simulink model "B2_IEEE_13_bus"  (R2022b)
settings: Solver=ode4  StartTime=0.0  StopTime=tend  FixedStep=ts  MaxStep=0.04  RelTol=1e-3
undefined symbols (not defined in the file): C, C_601, C_602, C_603, C_604, C_605, C_606, C_607, C_bc_ESS, C_bc_PV, C_bc_SC, C_SC_set, Cf, f0, fc, fc1, ft2km, fv, Gf, Idcbase, Ilim, J, Ki_c1, Ki_v, Kp_c1, Kp_v, L_601, L_602, L_603, L_604, L_605, L_606, L_607, L_bc_ESS, L_bc_PV, L_bc_SC, L_line_ESS, L_line_PV, Lf, Pnom, Pset_ESS, Pset_inv, Pset_load, Pset_PV, Pset_SC, Qset_inv, R_601, R_602, R_603, R_604, R_605, R_606, R_607, R_bc_ESS, R_bc_PV, R_bc_SC, R_line_ESS, R_line_PV, R_line_SC, Rf ... (+23)
libraries: spsSeriesRLCBranchLib x12, spsLoadFlowBusLib x12, spsPiSectionLineLib x9, spsThreePhaseVIMeasurementLib x8, spsVoltageMeasurementLib x8, cstblocks x8, spsThreePhaseSeriesRLCLoadLib x7, spsCurrentMeasurementLib x6, simulink_extras x6, spsGroundLib x6, spsMultimeterLib x6, spsPowerLib x6
(part 2 of 2)

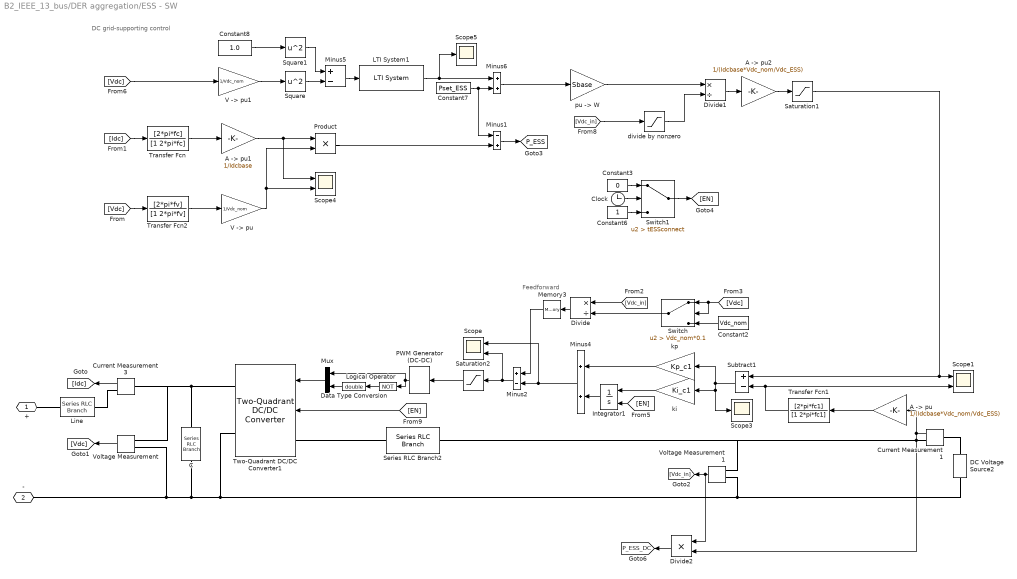
== system B2_IEEE_13_bus/DER aggregation/ESS - SW ==
  note: Feedforward
  note: DC grid-supporting control
  "A -> pu" : Gain  Gain=1/(Idcbase*Vdc_nom/Vdc_ESS)
  "A -> pu1" : Gain  Gain=1/Idcbase
  "A -> pu2" : Gain  Gain=1/(Idcbase*Vdc_nom/Vdc_ESS)
  C : spsSeriesRLCBranchLib/Series RLC Branch  LConnTagsString=__new0  RConnTagsString=__new0  BranchType=C  Resistance=0.001  Inductance=L_line_PV  SetiL0=off  InitialCurrent=0  Capacitance=C_bc_ESS  Setx0=on  InitialVoltage=Vdc_nom  Measurements=None
  Clock : Clock
  Constant2 : Constant  Value=Vdc_nom
  Constant3 : Constant  Value=0
  Constant6 : Constant
  Constant7 : Constant  Value=Pset_ESS
  Constant8 : Constant  Value=1.0
  Current Measurement1 : spsCurrentMeasurementLib/Current Measurement  PhasorSimulation=off  OutputType=Complex  PSBequivalent=0
  Current Measurement3 : spsCurrentMeasurementLib/Current Measurement  PhasorSimulation=off  OutputType=Complex  PSBequivalent=0
  DC Voltage Source2 : spsDCVoltageSourceLib/DC Voltage Source  Amplitude=Vdc_ESS  Measurements=None
  Data Type Conversion : DataTypeConversion  OutDataTypeStr=double  SaturateOnIntegerOverflow=off  RndMeth=Floor
  Divide : Product  Inputs=*/
  Divide1 : Product  Inputs=*/
  Divide2 : Product  Inputs=**
  Integrator1 : Integrator  ExternalReset=level hold  LimitOutput=on  UpperSaturationLimit=1  LowerSaturationLimit=-1
  LTI System1 : cstblocks/LTI System  sys=T_ESS1  IC=[]
  Line : spsSeriesRLCBranchLib/Series RLC Branch  LConnTagsString=__new0  RConnTagsString=__new0  BranchType=R  Resistance=R_line_ESS  Inductance=L_line_ESS  SetiL0=off  InitialCurrent=0  Capacitance=1e-6  Setx0=off  InitialVoltage=0  Measurements=None
  Logical Operator : Logic  Operator=NOT  AllPortsSameDT=off  OutDataTypeStr=boolean
  Memory3 : Memory
  Minus1 : Sum  Inputs=-+
  Minus2 : Sum  Inputs=+-
  Minus4 : Sum
  Minus5 : Sum  Inputs=+-
  Minus6 : Sum
  Mux : Mux  Inputs=2
  PWM Generator (DC-DC) : spsPWMGeneratorDCDCLib/PWM Generator (DC-DC)  Fsw=fw  Ts=0
  Product : Product
  Saturation1 : Saturate  UpperLimit=1.0  LowerLimit=-1.0
  Saturation2 : Saturate  UpperLimit=1  LowerLimit=0
  Scope : Scope  NumInputPorts=2
  Scope1 : Scope  NumInputPorts=2
  Scope3 : Scope
  Scope4 : Scope  NumInputPorts=2
  Scope5 : Scope
  Series RLC Branch2 : spsSeriesRLCBranchLib/Series RLC Branch  LConnTagsString=__new0  RConnTagsString=__new0  BranchType=RL  Resistance=R_bc_ESS  Inductance=L_bc_ESS  SetiL0=off  InitialCurrent=Pset_ESS*Idcbase*Vdc_nom/Vdc_PV  Capacitance=1e-6  Setx0=off  InitialVoltage=0  Measurements=None
  Square : Math  Operator=square
  Square1 : Math  Operator=square
  Subtract1 : Sum  Inputs=+-
  Switch : Switch  Criteria=u2 > Threshold  Threshold=Vdc_nom*0.1  SaturateOnIntegerOverflow=off  InputSameDT=off
  Switch1 : Switch  Criteria=u2 > Threshold  Threshold=tESSconnect  SaturateOnIntegerOverflow=off  InputSameDT=off
  Transfer Fcn : TransferFcn  Numerator=[2*pi*fc]  Denominator=[1 2*pi*fc]
  Transfer Fcn1 : TransferFcn  Numerator=[2*pi*fc1]  Denominator=[1 2*pi*fc1]
  Transfer Fcn2 : TransferFcn  Numerator=[2*pi*fv]  Denominator=[1 2*pi*fv]
  Two-Quadrant DC/DC Converter1 : spsTwoQuadrantDCDCConverterLib/Two-Quadrant DC//DC Converter  ModelType=Switching devices  Ron=1e-4  Rs=1e6  Cs=inf  Vforward=[0,0]  Ron_Diode=1e-3  Rs_Diode=1e6  Cs_Diode=inf  Vf_Diode=1e-3  Rs_CurrentSource=inf  Ron_ACsource=1e-3
      settings: LibrarySourceBlock=|
      | sps_lib/Power Electronics/Two-Quadrant
      | DC//DC Converter
  "V -> pu" : Gain  Gain=1/Vdc_nom
  "V -> pu1" : Gain  Gain=1/Vdc_nom
  Voltage Measurement : spsVoltageMeasurementLib/Voltage Measurement  PhasorSimulation=off  OutputType=Complex  PSBequivalent=0
  Voltage Measurement1 : spsVoltageMeasurementLib/Voltage Measurement  PhasorSimulation=off  OutputType=Complex  PSBequivalent=0
  divide by nonzero : Saturate  UpperLimit=1e6  LowerLimit=1e-6
  ki : Gain  Gain=Ki_c1
  kp : Gain  Gain=Kp_c1
  "pu -> W" : Gain  Gain=Sbase
  + : PMIOPort  Side=Left
  - : PMIOPort  Port=2  Side=Right
  tag scope: P_ESS=global, P_ESS_DC=global
  wires:
  Constant6/1 -> Switch1/3
  Switch1/1 -> [EN]
  Clock/1 -> Switch1/2
  Constant3/1 -> Switch1/1
  Minus6/1 -> "pu -> W"/1
  Saturation1/1 -> Scope1/1, Subtract1/1
  Divide1/1 -> "A -> pu2"/1
  "pu -> W"/1 -> Divide1/1
  divide by nonzero/1 -> Divide1/2
  Subtract1/1 -> Scope3/1, ki/1, kp/1
  Memory3/1 -> Minus2/1
  Transfer Fcn2/1 -> "V -> pu"/1
  Transfer Fcn/1 -> "A -> pu1"/1
  Minus2/1 -> Scope/2, Saturation2/1
  Minus4/1 -> Minus2/2, Scope/1
  [Vdc] -> Transfer Fcn2/1
  "A -> pu1"/1 -> Product/1, Scope4/1
  "V -> pu"/1 -> Scope4/2, Product/2
  "V -> pu1"/1 -> Square/1
  [Vdc] -> "V -> pu1"/1
  LTI System1/1 -> Scope5/1, Minus6/1
  Constant7/1 -> Minus6/2, Minus1/1
  Minus5/1 -> LTI System1/1
  Square1/1 -> Minus5/1
  Square/1 -> Minus5/2
  Constant8/1 -> Square1/1
  [EN] -> Integrator1/2
  ki/1 -> Integrator1/1
  Integrator1/1 -> Minus4/2
  kp/1 -> Minus4/1
  "A -> pu2"/1 -> Saturation1/1
  [Vdc] -> Switch/1, Switch/2
  Divide/1 -> Memory3/1
  [Vdc_in] -> Divide/1
  Constant2/1 -> Switch/3
  Switch/1 -> Divide/2
  Product/1 -> Minus1/2
  Transfer Fcn1/1 -> Subtract1/2, Scope1/2
  [EN] -> Two-Quadrant DC/DC Converter1/2
  Current Measurement3/1 -> [Idc]
  Voltage Measurement/1 -> [Vdc]
  [Idc] -> Transfer Fcn/1
  "A -> pu"/1 -> Transfer Fcn1/1
  Minus1/1 -> [P_ESS]
  Saturation2/1 -> PWM Generator (DC-DC)/1
  PWM Generator (DC-DC)/1 -> Mux/1, Logical Operator/1
  Logical Operator/1 -> Data Type Conversion/1
  Data Type Conversion/1 -> Mux/2
  Mux/1 -> Two-Quadrant DC/DC Converter1/1
  [Vdc_in] -> divide by nonzero/1
  Voltage Measurement1/1 -> Divide2/1, [Vdc_in]
  Current Measurement1/1 -> "A -> pu"/1, Divide2/2
  Divide2/1 -> [P_ESS_DC]
  connections:
  Line/LConn1 -- +/RConn1
  C/LConn1 -- Two-Quadrant DC/DC Converter1/RConn1 -- Voltage Measurement/LConn1 -- Current Measurement3/LConn1
  Current Measurement3/RConn1 -- Line/RConn1
  Current Measurement1/RConn1 -- Voltage Measurement1/LConn1 -- Series RLC Branch2/RConn1
  DC Voltage Source2/RConn1 -- Current Measurement1/LConn1
  Two-Quadrant DC/DC Converter1/LConn1 -- Series RLC Branch2/LConn1
  Voltage Measurement/LConn2 -- -/RConn1 -- C/RConn1 -- Two-Quadrant DC/DC Converter1/RConn2 -- DC Voltage Source2/LConn1 -- Voltage Measurement1/LConn2

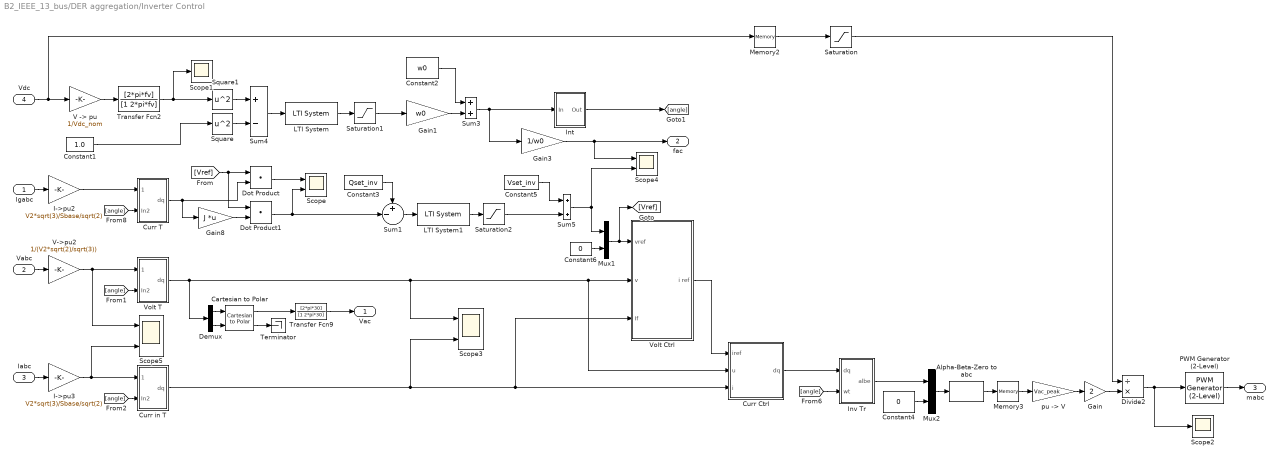
== system B2_IEEE_13_bus/DER aggregation/Inverter Control ==
  Igabc : Inport
  Vabc : Inport  Port=2
  Iabc : Inport  Port=3
  Vdc : Inport  Port=4
  Alpha-Beta-Zero to abc : spsAlphaBetaZerotoabcLib/Alpha-Beta-Zero to abc
  Cartesian to Polar : simulink_extras/Transformations/Cartesian to Polar
  Constant1 : Constant  Value=1.0
  Constant2 : Constant  Value=w0
  Constant3 : Constant  Value=Qset_inv
  Constant4 : Constant  Value=0
  Constant5 : Constant  Value=Vset_inv
  Constant6 : Constant  Value=0
  Curr Ctrl : Subsystem
  Curr T : Subsystem
  Curr in T : Subsystem
  Demux : Demux  Outputs=2
  Divide2 : Product  Inputs=/*
  Dot Product : DotProduct  OutDataTypeStr=Inherit: Inherit via internal rule
  Dot Product1 : DotProduct  OutDataTypeStr=Inherit: Inherit via internal rule
  Gain : Gain  Gain=2
  Gain1 : Gain  Gain=w0
  Gain3 : Gain  Gain=1/w0
  Gain8 : Gain  Gain=J  Multiplication=Matrix(K*u)
  I->pu2 : Gain  Gain=V2*sqrt(3)/Sbase/sqrt(2)  SaturateOnIntegerOverflow=on  OutDataTypeStr=Inherit: Same as input  ParamDataTypeStr=Inherit: Same as input
  I->pu3 : Gain  Gain=V2*sqrt(3)/Sbase/sqrt(2)  SaturateOnIntegerOverflow=on  OutDataTypeStr=Inherit: Same as input  ParamDataTypeStr=Inherit: Same as input
  Int : Subsystem
  Inv Tr : Subsystem
  LTI System : cstblocks/LTI System  sys=T_des_fvdc  IC=[]
  LTI System1 : cstblocks/LTI System  sys=T_des_vq  IC=[]
  Memory2 : Memory
  Memory3 : Memory
  Mux1 : Mux  Inputs=2
  Mux2 : Mux  Inputs=2
  PWM Generator (2-Level) : spsPWMGenerator2LevelLib/PWM Generator (2-Level)  ModulatorType=Three-phase bridge (6 pulses)  ModulatorMode=Unsynchronized  Fc=fw  Pc=90  nF=27  MinMax="[ -1  1 ]"  SamplingTechnique=Natural  ModulatingSignals=off  m=0.8  Freq=60  Phase=0  Ts=0  ShowCarrierOutport=off
  Saturation : Saturate  UpperLimit=Vdc_nom*1.1  LowerLimit=Vdc_nom*0.9
  Saturation1 : Saturate  UpperLimit=0.1  LowerLimit=-0.1
  Saturation2 : Saturate
  Scope{,3..5} (4 alike) : Scope  NumInputPorts=2
  Scope1 : Scope
  Scope2 : Scope
  Square : Math  Operator=square
  Square1 : Math  Operator=square
  Sum1 : Sum  Inputs=+-|
  Sum3 : Sum
  Sum4 : Sum  Inputs=+-
  Sum5 : Sum
  Terminator : Terminator
  Transfer Fcn2 : TransferFcn  Numerator=[2*pi*fv]  Denominator=[1 2*pi*fv]
  Transfer Fcn9 : TransferFcn  Numerator=[2*pi*30]  Denominator=[1 2*pi*30]
  "V -> pu" : Gain  Gain=1/Vdc_nom
  V->pu2 : Gain  Gain=1/(V2*sqrt(2)/sqrt(3))  SaturateOnIntegerOverflow=on  OutDataTypeStr=Inherit: Same as input  ParamDataTypeStr=Inherit: Same as input
  Volt Ctrl : Subsystem
  Volt T : Subsystem
  "pu -> V" : Gain  Gain=Vac_peak
  Vac : Outport
  fac : Outport  Port=2
  mabc : Outport  Port=3
  wires:
  Transfer Fcn9/1 -> Vac/1
  Memory3/1 -> "pu -> V"/1
  Curr Ctrl/1(dq) -> Inv Tr/1(dq)
  Mux1/1 -> Volt Ctrl/1(vref), [Vref]
  Constant6/1 -> Mux1/2
  Sum5/1 -> Mux1/1, Scope4/2
  Cartesian to Polar/1 -> Transfer Fcn9/1
  Cartesian to Polar/2 -> Terminator/1
  Demux/1 -> Cartesian to Polar/1
  Demux/2 -> Cartesian to Polar/2
  Int/1(Out) -> [angle]
  Inv Tr/1(albe) -> Mux2/1
  [angle] -> Inv Tr/2(wt)
  Volt Ctrl/1(i ref) -> Curr Ctrl/1(iref)
  Curr in T/1(dq) -> Curr Ctrl/3(i), Volt Ctrl/3(If), Scope3/2
  Volt T/1(dq) -> Scope3/1, Volt Ctrl/2(v), Curr Ctrl/2("u "), Demux/1
  Gain8/1 -> Dot Product1/2
  Curr T/1(dq) -> Gain8/1, Dot Product/2
  [Vref] -> Dot Product1/1, Dot Product/1
  [angle] -> Curr in T/2(In2)
  I->pu3/1 -> Curr in T/1(abc), Scope5/2
  V->pu2/1 -> Volt T/1(abc), Scope5/1
  [angle] -> Volt T/2(In2)
  [angle] -> Curr T/2(In2)
  I->pu2/1 -> Curr T/1(abc)
  Iabc/1 -> I->pu3/1
  PWM Generator (2-Level)/1 -> mabc/1
  Transfer Fcn2/1 -> Square1/1, Scope1/1
  Saturation1/1 -> Gain1/1
  Memory2/1 -> Saturation/1
  "V -> pu"/1 -> Transfer Fcn2/1
  Vdc/1 -> Memory2/1, "V -> pu"/1
  Saturation/1 -> Divide2/1
  Saturation2/1 -> Sum5/2
  LTI System/1 -> Saturation1/1
  Gain3/1 -> fac/1, Scope4/1
  Square1/1 -> Sum4/1
  Square/1 -> Sum4/2
  Constant3/1 -> Sum1/1
  Sum1/1 -> LTI System1/1
  Divide2/1 -> PWM Generator (2-Level)/1, Scope2/1
  "pu -> V"/1 -> Gain/1
  Dot Product1/1 -> Sum1/2, Scope/2
  Dot Product/1 -> Scope/1
  Constant1/1 -> Square/1
  Constant5/1 -> Sum5/1
  Mux2/1 -> Alpha-Beta-Zero to abc/1
  Gain1/1 -> Sum3/2
  Constant4/1 -> Mux2/2
  Sum4/1 -> LTI System/1
  LTI System1/1 -> Saturation2/1
  Constant2/1 -> Sum3/1
  Alpha-Beta-Zero to abc/1 -> Memory3/1
  Sum3/1 -> Gain3/1, Int/1(In)
  Gain/1 -> Divide2/2
  Vabc/1 -> V->pu2/1
  Igabc/1 -> I->pu2/1

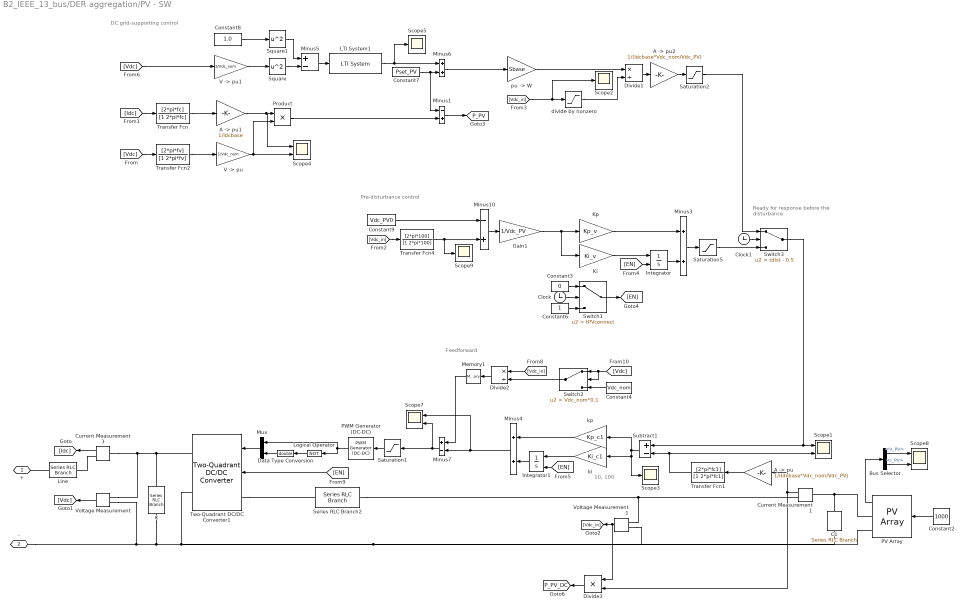
== system B2_IEEE_13_bus/DER aggregation/PV - SW ==
  note: Ready for response
      | before the disturbance
  note: Feedforward
  note: DC grid-supporting control
  note: 10, 100
  note: Pre-disturbance control
  "A -> pu" : Gain  Gain=1/(Idcbase*Vdc_nom/Vdc_PV)
  "A -> pu1" : Gain  Gain=1/Idcbase
  "A -> pu2" : Gain  Gain=1/(Idcbase*Vdc_nom/Vdc_PV)
  Bus Selector : BusSelector  OutputSignals=V_PV,I_PV
  C : spsSeriesRLCBranchLib/Series RLC Branch  LConnTagsString=__new0  RConnTagsString=__new0  BranchType=C  Resistance=0.001  Inductance=L_line_PV  SetiL0=off  InitialCurrent=0  Capacitance=C_bc_PV  Setx0=on  InitialVoltage=Vdc_nom  Measurements=None
  C1 : spsSeriesRLCBranchLib/Series RLC Branch  LConnTagsString=__new0  RConnTagsString=__new0  BranchType=C  Resistance=0.001  Inductance=L_line_PV  SetiL0=off  InitialCurrent=0  Capacitance=C_bc_PV  Setx0=on  InitialVoltage=Vdc_PV0  Measurements=None
  Clock : Clock
  Clock1 : Clock
  Constant2 : Constant  Value=1000
  Constant3 : Constant  Value=0
  Constant4 : Constant  Value=Vdc_nom
  Constant6 : Constant
  Constant7 : Constant  Value=Pset_PV
  Constant8 : Constant  Value=1.0
  Constant9 : Constant  Value=Vdc_PV0
  Current Measurement1 : spsCurrentMeasurementLib/Current Measurement  PhasorSimulation=off  OutputType=Complex  PSBequivalent=0
  Current Measurement3 : spsCurrentMeasurementLib/Current Measurement  PhasorSimulation=off  OutputType=Complex  PSBequivalent=0
  Data Type Conversion : DataTypeConversion  OutDataTypeStr=double  SaturateOnIntegerOverflow=off  RndMeth=Floor
  Divide1 : Product  Inputs=*/
  Divide2 : Product  Inputs=*/
  Divide3 : Product  Inputs=**
  Gain1 : Gain  Gain=1/Vdc_PV
  Integrator : Integrator  ExternalReset=level hold  UpperSaturationLimit=1.5  LowerSaturationLimit=-0.5
  Integrator1 : Integrator  ExternalReset=level hold  LimitOutput=on  UpperSaturationLimit=1  LowerSaturationLimit=-1
  Ki : Gain  Gain=Ki_v
  Kp : Gain  Gain=Kp_v
  LTI System1 : cstblocks/LTI System  sys=T_PV  IC=[]
  Line : spsSeriesRLCBranchLib/Series RLC Branch  LConnTagsString=__new0  RConnTagsString=__new0  BranchType=R  Resistance=R_line_PV  Inductance=L_line_PV  SetiL0=off  InitialCurrent=0  Capacitance=1e-6  Setx0=off  InitialVoltage=0  Measurements=None
  Logical Operator : Logic  Operator=NOT  AllPortsSameDT=off  OutDataTypeStr=boolean
  Memory1 : Memory
  Minus1 : Sum  Inputs=-+
  Minus10 : Sum  Inputs=-+
  Minus3 : Sum
  Minus4 : Sum
  Minus5 : Sum  Inputs=+-
  Minus6 : Sum
  Minus7 : Sum  Inputs=+-
  Mux : Mux  Inputs=2
  PV Array : spsPVArrayLib/PV Array  Npar=291  Nser=8  PlotType=array @ 1000 W/m2 & specified temperatures  S_vec="[ 1000  500  100 ]"  Temp_C_vec=40  ModuleName=SunPower SPR-315E-WHT-D  PlotWhenSelected=off  Pm=315.072  Ncell=96  Voc=64.6  Isc=6.14  Vm=54.7  Im=5.76  beta_Voc_pc=-0.2727  alpha_Isc_pc=0.061743  beta_Voc=-0.17616  alpha_Isc=0.003791  IL=6.1461  I0=6.5067e-12  nI=0.95071  Rsh=430.0666  Rs=0.43041  RobustModel=on  RobustCellTemperature=40  BAL=off  Tc=1e-6  Tfilter=5e-5
  PWM Generator (DC-DC) : spsPWMGeneratorDCDCLib/PWM Generator (DC-DC)  Fsw=fw  Ts=0
  Product : Product
  Saturation1 : Saturate  UpperLimit=1  LowerLimit=0
  Saturation2 : Saturate  UpperLimit=1.0  LowerLimit=-1.0
  Saturation5 : Saturate  UpperLimit=1.0  LowerLimit=-1.0
  Scope{1,4,7..8} (4 alike) : Scope  NumInputPorts=2
  Scope{2..3,5,9} (4 alike) : Scope
  Series RLC Branch2 : spsSeriesRLCBranchLib/Series RLC Branch  LConnTagsString=__new0  RConnTagsString=__new0  BranchType=RL  Resistance=R_bc_PV  Inductance=L_bc_PV  SetiL0=off  InitialCurrent=Pset_PV*Idcbase*Vdc_nom/Vdc_PV  Capacitance=1e-6  Setx0=off  InitialVoltage=0  Measurements=None
  Square : Math  Operator=square
  Square1 : Math  Operator=square
  Subtract1 : Sum  Inputs=+-
  Switch1 : Switch  Criteria=u2 > Threshold  Threshold=tPVconnect  SaturateOnIntegerOverflow=off  InputSameDT=off
  Switch2 : Switch  Criteria=u2 > Threshold  Threshold=Vdc_nom*0.1  SaturateOnIntegerOverflow=off  InputSameDT=off
  Switch3 : Switch  Criteria=u2 > Threshold  Threshold=tdist - 0.5  SaturateOnIntegerOverflow=off  InputSameDT=off
  Transfer Fcn : TransferFcn  Numerator=[2*pi*fc]  Denominator=[1 2*pi*fc]
  Transfer Fcn1 : TransferFcn  Numerator=[2*pi*fc1]  Denominator=[1 2*pi*fc1]
  Transfer Fcn2 : TransferFcn  Numerator=[2*pi*fv]  Denominator=[1 2*pi*fv]
  Transfer Fcn4 : TransferFcn  Numerator=[2*pi*100]  Denominator=[1 2*pi*100]
  Two-Quadrant DC/DC Converter1 : spsTwoQuadrantDCDCConverterLib/Two-Quadrant DC//DC Converter  ModelType=Switching devices  Ron=1e-4  Rs=1e6  Cs=inf  Vforward=[0,0]  Ron_Diode=1e-3  Rs_Diode=1e6  Cs_Diode=inf  Vf_Diode=1e-3  Rs_CurrentSource=inf  Ron_ACsource=1e-3
      settings: LibrarySourceBlock=|
      | sps_lib/Power Electronics/Two-Quadrant
      | DC//DC Converter
  "V -> pu" : Gain  Gain=1/Vdc_nom
  "V -> pu1" : Gain  Gain=1/Vdc_nom
  Voltage Measurement : spsVoltageMeasurementLib/Voltage Measurement  PhasorSimulation=off  OutputType=Complex  PSBequivalent=0
  Voltage Measurement1 : spsVoltageMeasurementLib/Voltage Measurement  PhasorSimulation=off  OutputType=Complex  PSBequivalent=0
  divide by nonzero : Saturate  UpperLimit=1e6  LowerLimit=1e-6
  ki : Gain  Gain=Ki_c1
  kp : Gain  Gain=Kp_c1
  "pu -> W" : Gain  Gain=Sbase
  + : PMIOPort  Side=Left
  - : PMIOPort  Port=2  Side=Right
  tag scope: P_PV=global, P_PV_DC=global
  wires:
  Minus4/1 -> Minus7/2, Scope7/1
  Clock/1 -> Switch1/2
  Constant3/1 -> Switch1/1
  Constant6/1 -> Switch1/3
  Switch1/1 -> [EN]
  Saturation2/1 -> Switch3/1
  Saturation5/1 -> Switch3/3
  Clock1/1 -> Switch3/2
  Minus1/1 -> [P_PV]
  Minus6/1 -> "pu -> W"/1
  Divide1/1 -> "A -> pu2"/1
  divide by nonzero/1 -> Divide1/2
  "pu -> W"/1 -> Divide1/1
  "A -> pu2"/1 -> Saturation2/1
  Transfer Fcn4/1 -> Minus10/2, Scope9/1
  [Vdc_in] -> Transfer Fcn4/1
  Minus10/1 -> Gain1/1
  Constant9/1 -> Minus10/1
  Constant2/1 -> PV Array/1
  Bus Selector/2 -> Scope8/2  "<I_PV>"
  Bus Selector/1 -> Scope8/1  "<V_PV>"
  PV Array/1 -> Bus Selector/1
  Minus7/1 -> Saturation1/1, Scope7/2
  Memory1/1 -> Minus7/1
  Divide2/1 -> Memory1/1
  Switch3/1 -> Subtract1/1, Scope1/1
  [Vdc_in] -> Divide2/1
  [Vdc] -> Switch2/1, Switch2/2
  Constant4/1 -> Switch2/3
  Switch2/1 -> Divide2/2
  [Idc] -> Transfer Fcn/1
  Voltage Measurement/1 -> [Vdc]
  Current Measurement3/1 -> [Idc]
  [EN] -> Two-Quadrant DC/DC Converter1/2
  Minus3/1 -> Saturation5/1
  Ki/1 -> Integrator/1
  Integrator/1 -> Minus3/2
  Kp/1 -> Minus3/1
  kp/1 -> Minus4/1
  Integrator1/1 -> Minus4/2
  ki/1 -> Integrator1/1
  Subtract1/1 -> kp/1, ki/1, Scope3/1
  [EN] -> Integrator/2
  [EN] -> Integrator1/2
  Constant8/1 -> Square1/1
  Square/1 -> Minus5/2
  Square1/1 -> Minus5/1
  Minus5/1 -> LTI System1/1
  Constant7/1 -> Minus6/2, Minus1/1
  LTI System1/1 -> Minus6/1, Scope5/1
  [Vdc] -> "V -> pu1"/1
  "V -> pu1"/1 -> Square/1
  "V -> pu"/1 -> Product/2, Scope4/2
  "A -> pu1"/1 -> Scope4/1, Product/1
  [Vdc] -> Transfer Fcn2/1
  Gain1/1 -> Kp/1, Ki/1
  Transfer Fcn/1 -> "A -> pu1"/1
  Transfer Fcn2/1 -> "V -> pu"/1
  Transfer Fcn1/1 -> Scope1/2, Subtract1/2
  "A -> pu"/1 -> Transfer Fcn1/1
  Logical Operator/1 -> Data Type Conversion/1
  Saturation1/1 -> PWM Generator (DC-DC)/1
  PWM Generator (DC-DC)/1 -> Mux/1, Logical Operator/1
  Data Type Conversion/1 -> Mux/2
  Product/1 -> Minus1/2
  Mux/1 -> Two-Quadrant DC/DC Converter1/1
  [Vdc_in] -> divide by nonzero/1, Scope2/1
  Voltage Measurement1/1 -> Divide3/1, [Vdc_in]
  Current Measurement1/1 -> "A -> pu"/1, Divide3/2
  Divide3/1 -> [P_PV_DC]
  connections:
  -/RConn1 -- Two-Quadrant DC/DC Converter1/RConn2 -- Voltage Measurement1/LConn2 -- PV Array/RConn2 -- C1/RConn1 -- C/RConn1 -- Voltage Measurement/LConn2
  Two-Quadrant DC/DC Converter1/LConn1 -- Series RLC Branch2/LConn1
  PV Array/RConn1 -- Current Measurement1/LConn1 -- C1/LConn1
  Voltage Measurement1/LConn1 -- Series RLC Branch2/RConn1 -- Current Measurement1/RConn1
  Current Measurement3/RConn1 -- Line/RConn1
  Two-Quadrant DC/DC Converter1/RConn1 -- C/LConn1 -- Current Measurement3/LConn1 -- Voltage Measurement/LConn1
  Line/LConn1 -- +/RConn1

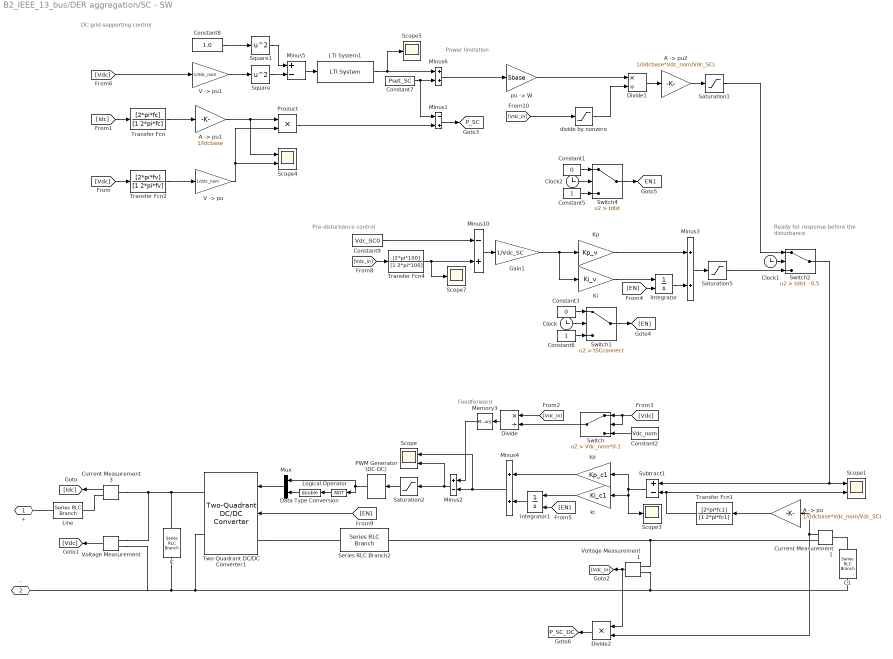
== system B2_IEEE_13_bus/DER aggregation/SC - SW ==
  note: Power limitation
  note: Pre-disturbance control
  note: DC grid-supporting control
  note: Feedforward
  note: Ready for response
      | before the disturbance
  "A -> pu" : Gain  Gain=1/(Idcbase*Vdc_nom/Vdc_SC)
  "A -> pu1" : Gain  Gain=1/Idcbase
  "A -> pu2" : Gain  Gain=1/(Idcbase*Vdc_nom/Vdc_SC)
  C : spsSeriesRLCBranchLib/Series RLC Branch  LConnTagsString=__new0  RConnTagsString=__new0  BranchType=C  Resistance=0.001  Inductance=L_line_PV  SetiL0=off  InitialCurrent=0  Capacitance=C_bc_SC  Setx0=on  InitialVoltage=Vdc_nom  Measurements=None
  C1 : spsSeriesRLCBranchLib/Series RLC Branch  LConnTagsString=__new0  RConnTagsString=__new0  BranchType=C  Resistance=0.001  Inductance=L_line_PV  SetiL0=off  InitialCurrent=0  Capacitance=C_SC_set  Setx0=on  InitialVoltage=Vdc_SC0  Measurements=None
  Clock : Clock
  Clock1 : Clock
  Clock2 : Clock
  Constant1 : Constant  Value=0
  Constant2 : Constant  Value=Vdc_nom
  Constant3 : Constant  Value=0
  Constant5 : Constant
  Constant6 : Constant
  Constant7 : Constant  Value=Pset_SC
  Constant8 : Constant  Value=1.0
  Constant9 : Constant  Value=Vdc_SC0
  Current Measurement1 : spsCurrentMeasurementLib/Current Measurement  PhasorSimulation=off  OutputType=Complex  PSBequivalent=0
  Current Measurement3 : spsCurrentMeasurementLib/Current Measurement  PhasorSimulation=off  OutputType=Complex  PSBequivalent=0
  Data Type Conversion : DataTypeConversion  OutDataTypeStr=double  SaturateOnIntegerOverflow=off  RndMeth=Floor
  Divide : Product  Inputs=*/
  Divide1 : Product  Inputs=*/
  Divide2 : Product  Inputs=**
  Gain1 : Gain  Gain=1/Vdc_SC
  Integrator : Integrator  ExternalReset=level hold  UpperSaturationLimit=1.5  LowerSaturationLimit=-0.5
  Integrator1 : Integrator  ExternalReset=level hold  LimitOutput=on  UpperSaturationLimit=1  LowerSaturationLimit=-1
  Ki : Gain  Gain=Ki_v
  Kp : Gain  Gain=Kp_v
  LTI System1 : cstblocks/LTI System  sys=T_SC1  IC=[]
  Line : spsSeriesRLCBranchLib/Series RLC Branch  LConnTagsString=__new0  RConnTagsString=__new0  BranchType=R  Resistance=R_line_SC  Inductance=L_line_ESS  SetiL0=off  InitialCurrent=0  Capacitance=1e-6  Setx0=off  InitialVoltage=0  Measurements=None
  Logical Operator : Logic  Operator=NOT  AllPortsSameDT=off  OutDataTypeStr=boolean
  Memory3 : Memory
  Minus1 : Sum  Inputs=-+
  Minus10 : Sum  Inputs=-+
  Minus2 : Sum  Inputs=+-
  Minus3 : Sum
  Minus4 : Sum
  Minus5 : Sum  Inputs=+-
  Minus6 : Sum
  Mux : Mux  Inputs=2
  PWM Generator (DC-DC) : spsPWMGeneratorDCDCLib/PWM Generator (DC-DC)  Fsw=fw  Ts=0
  Product : Product
  Saturation1 : Saturate  UpperLimit=1.0  LowerLimit=-1.0
  Saturation2 : Saturate  UpperLimit=1  LowerLimit=0
  Saturation5 : Saturate  UpperLimit=1.0  LowerLimit=-1.0
  Scope : Scope  NumInputPorts=2
  Scope1 : Scope  NumInputPorts=2
  Scope3 : Scope
  Scope4 : Scope  NumInputPorts=2
  Scope5 : Scope
  Scope7 : Scope
  Series RLC Branch2 : spsSeriesRLCBranchLib/Series RLC Branch  LConnTagsString=__new0  RConnTagsString=__new0  BranchType=RL  Resistance=R_bc_SC  Inductance=L_bc_SC  SetiL0=off  InitialCurrent=Pset_SC*Idcbase*Vdc_nom/Vdc_PV  Capacitance=1e-6  Setx0=off  InitialVoltage=0  Measurements=None
  Square : Math  Operator=square
  Square1 : Math  Operator=square
  Subtract1 : Sum  Inputs=+-
  Switch : Switch  Criteria=u2 > Threshold  Threshold=Vdc_nom*0.1  SaturateOnIntegerOverflow=off  InputSameDT=off
  Switch1 : Switch  Criteria=u2 > Threshold  Threshold=tSCconnect  SaturateOnIntegerOverflow=off  InputSameDT=off
  Switch2 : Switch  Criteria=u2 > Threshold  Threshold=tdist - 0.5  SaturateOnIntegerOverflow=off  InputSameDT=off
  Switch4 : Switch  Criteria=u2 > Threshold  Threshold=tdist  SaturateOnIntegerOverflow=off  InputSameDT=off
  Transfer Fcn : TransferFcn  Numerator=[2*pi*fc]  Denominator=[1 2*pi*fc]
  Transfer Fcn1 : TransferFcn  Numerator=[2*pi*fc1]  Denominator=[1 2*pi*fc1]
  Transfer Fcn2 : TransferFcn  Numerator=[2*pi*fv]  Denominator=[1 2*pi*fv]
  Transfer Fcn4 : TransferFcn  Numerator=[2*pi*100]  Denominator=[1 2*pi*100]
  Two-Quadrant DC/DC Converter1 : spsTwoQuadrantDCDCConverterLib/Two-Quadrant DC//DC Converter  ModelType=Switching devices  Ron=1e-4  Rs=1e6  Cs=inf  Vforward=[0,0]  Ron_Diode=1e-3  Rs_Diode=1e6  Cs_Diode=inf  Vf_Diode=1e-3  Rs_CurrentSource=inf  Ron_ACsource=1e-3
      settings: LibrarySourceBlock=|
      | sps_lib/Power Electronics/Two-Quadrant
      | DC//DC Converter
  "V -> pu" : Gain  Gain=1/Vdc_nom
  "V -> pu1" : Gain  Gain=1/Vdc_nom
  Voltage Measurement : spsVoltageMeasurementLib/Voltage Measurement  PhasorSimulation=off  OutputType=Complex  PSBequivalent=0
  Voltage Measurement1 : spsVoltageMeasurementLib/Voltage Measurement  PhasorSimulation=off  OutputType=Complex  PSBequivalent=0
  divide by nonzero : Saturate  UpperLimit=1e6  LowerLimit=1e-6
  ki : Gain  Gain=Ki_c1
  kp : Gain  Gain=Kp_c1
  "pu -> W" : Gain  Gain=Sbase
  + : PMIOPort  Side=Left
  - : PMIOPort  Port=2  Side=Right
  tag scope: EN1=global, P_SC=global, P_SC_DC=global
  wires:
  Constant1/1 -> Switch4/1
  Switch4/1 -> [EN1]
  Clock2/1 -> Switch4/2
  Constant5/1 -> Switch4/3
  Saturation5/1 -> Switch2/3
  Minus1/1 -> [P_SC]
  Minus6/1 -> "pu -> W"/1
  Subtract1/1 -> ki/1, Scope3/1, kp/1
  Divide1/1 -> "A -> pu2"/1
  divide by nonzero/1 -> Divide1/2
  "pu -> W"/1 -> Divide1/1
  "A -> pu2"/1 -> Saturation1/1
  Clock1/1 -> Switch2/2
  Minus10/1 -> Gain1/1
  [Vdc_in] -> Transfer Fcn4/1
  Constant9/1 -> Minus10/1
  Transfer Fcn4/1 -> Minus10/2, Scope7/1
  [Idc] -> Transfer Fcn/1
  Voltage Measurement/1 -> [Vdc]
  Current Measurement3/1 -> [Idc]
  [EN] -> Two-Quadrant DC/DC Converter1/2
  Current Measurement1/1 -> Divide2/2, "A -> pu"/1
  Transfer Fcn1/1 -> Subtract1/2, Scope1/2
  Product/1 -> Minus1/2
  Switch/1 -> Divide/2
  Constant2/1 -> Switch/3
  [Vdc_in] -> Divide/1
  Divide/1 -> Memory3/1
  Voltage Measurement1/1 -> Divide2/1, [Vdc_in]
  [Vdc] -> Switch/2, Switch/1
  Minus3/1 -> Saturation5/1
  Saturation1/1 -> Switch2/1
  Ki/1 -> Integrator/1
  Integrator/1 -> Minus3/2
  Kp/1 -> Minus3/1
  kp/1 -> Minus4/1
  Integrator1/1 -> Minus4/2
  ki/1 -> Integrator1/1
  Clock/1 -> Switch1/2
  Switch1/1 -> [EN]
  Constant3/1 -> Switch1/1
  Constant6/1 -> Switch1/3
  [EN] -> Integrator/2
  [EN] -> Integrator1/2
  Constant8/1 -> Square1/1
  Square/1 -> Minus5/2
  Square1/1 -> Minus5/1
  Minus5/1 -> LTI System1/1
  Constant7/1 -> Minus6/2, Minus1/1
  LTI System1/1 -> Minus6/1, Scope5/1
  [Vdc] -> "V -> pu1"/1
  "V -> pu1"/1 -> Square/1
  "V -> pu"/1 -> Product/2, Scope4/2
  "A -> pu1"/1 -> Scope4/1, Product/1
  [Vdc] -> Transfer Fcn2/1
  Minus4/1 -> Minus2/2, Scope/1
  Gain1/1 -> Kp/1, Ki/1
  Minus2/1 -> Scope/2, Saturation2/1
  Transfer Fcn/1 -> "A -> pu1"/1
  Transfer Fcn2/1 -> "V -> pu"/1
  "A -> pu"/1 -> Transfer Fcn1/1
  Memory3/1 -> Minus2/1
  Data Type Conversion/1 -> Mux/2
  Saturation2/1 -> PWM Generator (DC-DC)/1
  PWM Generator (DC-DC)/1 -> Mux/1, Logical Operator/1
  Logical Operator/1 -> Data Type Conversion/1
  Mux/1 -> Two-Quadrant DC/DC Converter1/1
  [Vdc_in] -> divide by nonzero/1
  Divide2/1 -> [P_SC_DC]
  Switch2/1 -> Subtract1/1, Scope1/1
  connections:
  C/RConn1 -- -/RConn1 -- Voltage Measurement/LConn2 -- Two-Quadrant DC/DC Converter1/RConn2 -- C1/RConn1 -- Voltage Measurement1/LConn2
  Two-Quadrant DC/DC Converter1/LConn1 -- Series RLC Branch2/LConn1
  C1/LConn1 -- Current Measurement1/LConn1
  Series RLC Branch2/RConn1 -- Voltage Measurement1/LConn1 -- Current Measurement1/RConn1
  Current Measurement3/RConn1 -- Line/RConn1
  Current Measurement3/LConn1 -- Voltage Measurement/LConn1 -- Two-Quadrant DC/DC Converter1/RConn1 -- C/LConn1
  Line/LConn1 -- +/RConn1

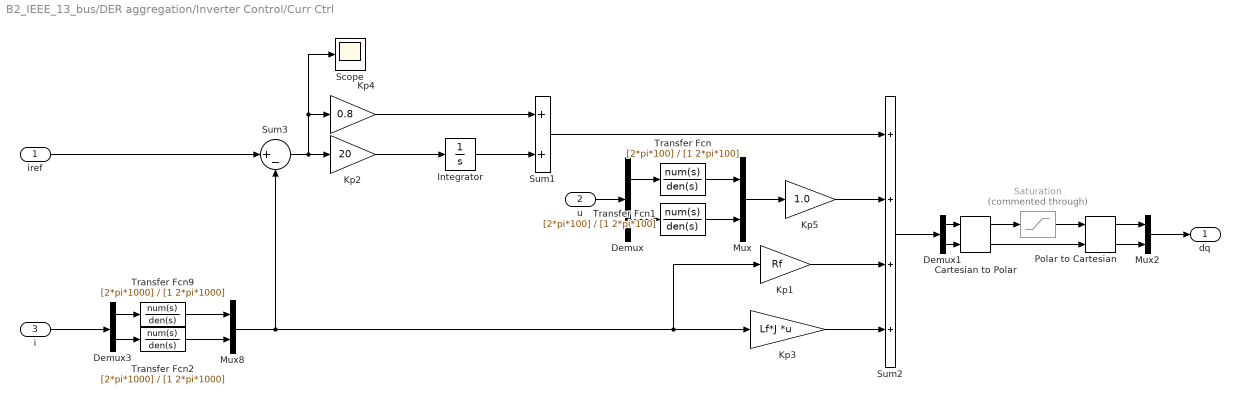
== system B2_IEEE_13_bus/DER aggregation/Inverter Control/Curr Ctrl ==
  iref : Inport
  "u " : Inport  Port=2
  i : Inport  Port=3
  Cartesian to Polar : simulink_extras/Transformations/Cartesian to Polar
  Demux : Demux  Outputs=2
  Demux1 : Demux  Outputs=2
  Demux3 : Demux  Outputs=2
  Integrator : Integrator  InitialCondition=[1 0]
  Kp1 : Gain  Gain=Rf  SaturateOnIntegerOverflow=on  OutDataTypeStr=Inherit: Same as input  ParamDataTypeStr=Inherit: Same as input
  Kp2 : Gain  Gain=20  SaturateOnIntegerOverflow=on  OutDataTypeStr=Inherit: Same as input  ParamDataTypeStr=Inherit: Same as input
  Kp3 : Gain  Gain=Lf*J  Multiplication=Matrix(K*u)  SaturateOnIntegerOverflow=on  OutDataTypeStr=Inherit: Same as input  ParamDataTypeStr=Inherit: Same as input
  Kp4 : Gain  Gain=0.8  SaturateOnIntegerOverflow=on  OutDataTypeStr=Inherit: Same as input  ParamDataTypeStr=Inherit: Same as input
  Kp5 : Gain  Gain=1.0  SaturateOnIntegerOverflow=on  OutDataTypeStr=Inherit: Same as input  ParamDataTypeStr=Inherit: Same as input
  Mux : Mux  Inputs=2
  Mux2 : Mux  Inputs=2
  Mux8 : Mux  Inputs=2
  Polar to Cartesian : simulink_extras/Transformations/Polar to Cartesian
  Saturation : Saturate  Commented=through  UpperLimit=1.5  LowerLimit=0
  Scope : Scope
  Sum1 : Sum
  Sum2 : Sum  Inputs=++++
  Sum3 : Sum  Inputs=|+-
  Transfer Fcn : TransferFcn  Numerator=[2*pi*100]  Denominator=[1 2*pi*100]
  Transfer Fcn1 : TransferFcn  Numerator=[2*pi*100]  Denominator=[1 2*pi*100]
  Transfer Fcn2 : TransferFcn  Numerator=[2*pi*1000]  Denominator=[1 2*pi*1000]
  Transfer Fcn9 : TransferFcn  Numerator=[2*pi*1000]  Denominator=[1 2*pi*1000]
  dq : Outport
  wires:
  Demux3/2 -> Transfer Fcn2/1
  i/1 -> Demux3/1
  Demux3/1 -> Transfer Fcn9/1
  Transfer Fcn9/1 -> Mux8/1
  Transfer Fcn2/1 -> Mux8/2
  iref/1 -> Sum3/1
  Saturation/1 -> Polar to Cartesian/1
  Polar to Cartesian/1 -> Mux2/1
  Sum2/1 -> Demux1/1
  Demux1/1 -> Cartesian to Polar/1
  Cartesian to Polar/1 -> Saturation/1
  Cartesian to Polar/2 -> Polar to Cartesian/2
  Polar to Cartesian/2 -> Mux2/2
  Demux1/2 -> Cartesian to Polar/2
  Transfer Fcn/1 -> Mux/1
  Transfer Fcn1/1 -> Mux/2
  Demux/2 -> Transfer Fcn1/1
  Demux/1 -> Transfer Fcn/1
  Mux/1 -> Kp5/1
  Kp5/1 -> Sum2/2
  "u "/1 -> Demux/1
  Kp3/1 -> Sum2/4
  Kp1/1 -> Sum2/3
  Mux2/1 -> dq/1
  Kp2/1 -> Integrator/1
  Mux8/1 -> Kp3/1, Kp1/1, Sum3/2
  Integrator/1 -> Sum1/2
  Kp4/1 -> Sum1/1
  Sum3/1 -> Kp2/1, Kp4/1, Scope/1
  Sum1/1 -> Sum2/1

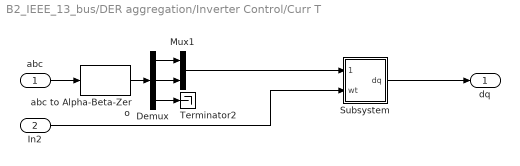
== system B2_IEEE_13_bus/DER aggregation/Inverter Control/Curr T ==
  abc : Inport
  In2 : Inport  Port=2
  Demux : Demux  Outputs=3
  Mux1 : Mux  Inputs=2
  Subsystem : Subsystem
  Terminator2 : Terminator
  abc to Alpha-Beta-Zero : spsabctoAlphaBetaZeroLib/abc to Alpha-Beta-Zero
  dq : Outport
  wires:
  In2/1 -> Subsystem/2(wt)
  Mux1/1 -> Subsystem/1(albe)
  abc/1 -> abc to Alpha-Beta-Zero/1
  Demux/2 -> Mux1/2
  Demux/1 -> Mux1/1
  Demux/3 -> Terminator2/1
  abc to Alpha-Beta-Zero/1 -> Demux/1
  Subsystem/1(dq) -> dq/1

== system B2_IEEE_13_bus/DER aggregation/Inverter Control/Curr in T ==
  abc : Inport
  In2 : Inport  Port=2
  Demux : Demux  Outputs=3
  Mux1 : Mux  Inputs=2
  Subsystem : Subsystem
  Terminator2 : Terminator
  abc to Alpha-Beta-Zero : spsabctoAlphaBetaZeroLib/abc to Alpha-Beta-Zero
  dq : Outport
  wires:
  Subsystem/1(dq) -> dq/1
  In2/1 -> Subsystem/2(wt)
  Mux1/1 -> Subsystem/1(albe)
  abc/1 -> abc to Alpha-Beta-Zero/1
  Demux/2 -> Mux1/2
  Demux/1 -> Mux1/1
  Demux/3 -> Terminator2/1
  abc to Alpha-Beta-Zero/1 -> Demux/1

== system B2_IEEE_13_bus/DER aggregation/Inverter Control/Int ==
  In : Inport
  Constant6 : Constant  Value=2*pi
  Initial : InitialCondition  Value=0
  Integrator1 : Integrator  ExternalReset=rising  InitialConditionSource=external  InitialCondition=sps.Phase_Init*pi/180  ShowStatePort=on
  Relational Operator : RelationalOperator  Operator=>  OutDataTypeStr=boolean  InputSameDT=off
  Subtract : Sum  Inputs=+-
  Out : Outport
  wires:
  Integrator1/1 -> Out/1
  Initial/1 -> Integrator1/3
  In/1 -> Integrator1/1
  Relational Operator/1 -> Integrator1/2
  Subtract/1 -> Initial/1
  Integrator1/State -> Relational Operator/1, Subtract/1
  Constant6/1 -> Relational Operator/2, Subtract/2

== system B2_IEEE_13_bus/DER aggregation/Inverter Control/Inv Tr ==
  dq : Inport
  wt : Inport  Port=2
  Fcn : Fcn  Expr=u[1]*cos(u[3]) - u[2]*sin(u[3])
  Fcn1 : Fcn  Expr=u[1]*sin(u[3]) + u[2]*cos(u[3])
  Mux : Mux  Inputs=2
  Mux2 : Mux  Inputs=[2 1]
  Mux3 : Mux  Inputs=[2 1]
  albe : Outport
  wires:
  Fcn1/1 -> Mux/2
  wt/1 -> Mux2/2, Mux3/2
  Fcn/1 -> Mux/1
  Mux/1 -> albe/1
  dq/1 -> Mux2/1, Mux3/1
  Mux2/1 -> Fcn/1
  Mux3/1 -> Fcn1/1

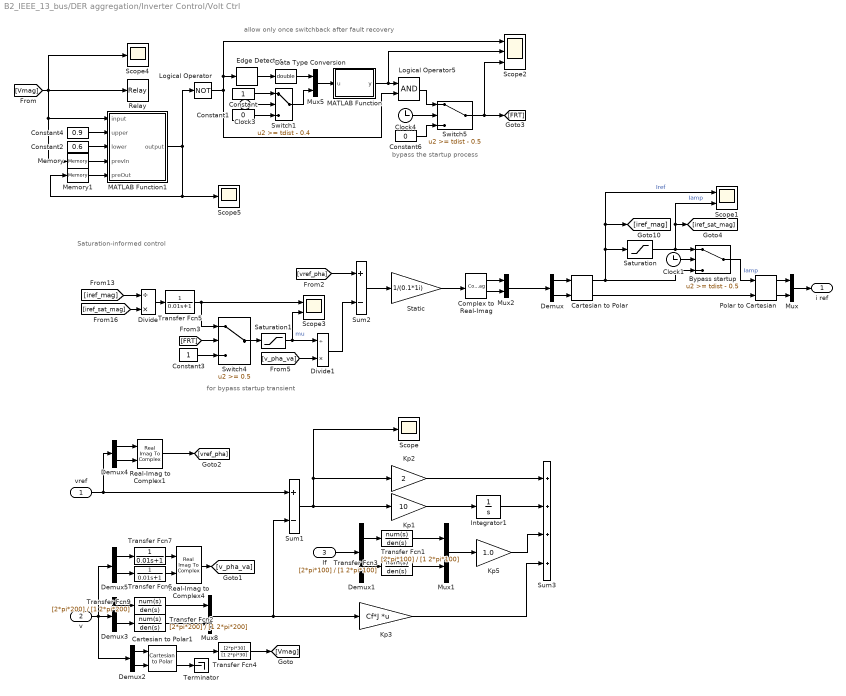
== system B2_IEEE_13_bus/DER aggregation/Inverter Control/Volt Ctrl ==
  note: Saturation-informed control
  note: for bypass startup transient
  note: bypass the startup process
  note: allow only once switchback after fault recovery
  vref : Inport
  v : Inport  Port=2
  If : Inport  Port=3
  Bypass startup : Switch  Threshold=tdist - 0.5  SaturateOnIntegerOverflow=off  InputSameDT=off
  Cartesian to Polar : simulink_extras/Transformations/Cartesian to Polar
  Cartesian to Polar1 : simulink_extras/Transformations/Cartesian to Polar
  Clock1 : Clock
  Clock3 : Clock
  Clock4 : Clock
  Complex to Real-Imag : ComplexToRealImag
  Constant : Constant
  Constant1 : Constant  Value=0
  Constant2 : Constant  Value=0.6
  Constant3 : Constant
  Constant4 : Constant  Value=0.9
  Constant6 : Constant  Value=0
  Data Type Conversion : DataTypeConversion  OutDataTypeStr=double  SaturateOnIntegerOverflow=off  RndMeth=Floor
  Demux{,1..5} (6 alike) : Demux  Outputs=2
  Divide : Product  Inputs=/*
  Divide1 : Product  Inputs=/*
  Edge Detector : spsEdgeDetectorLib/Edge Detector  model=Falling  ic=0  Ts=-1
      settings: LibrarySourceBlock=sps_lib/Control/Edge Detector
  Integrator1 : Integrator  InitialCondition=[0 0]
  Kp1 : Gain  Gain=10  SaturateOnIntegerOverflow=on  OutDataTypeStr=Inherit: Same as input  ParamDataTypeStr=Inherit: Same as input
  Kp2 : Gain  Gain=2  SaturateOnIntegerOverflow=on  OutDataTypeStr=Inherit: Same as input  ParamDataTypeStr=Inherit: Same as input
  Kp3 : Gain  Gain=Cf*J  Multiplication=Matrix(K*u)  SaturateOnIntegerOverflow=on  OutDataTypeStr=Inherit: Same as input  ParamDataTypeStr=Inherit: Same as input
  Kp5 : Gain  Gain=1.0  SaturateOnIntegerOverflow=on  OutDataTypeStr=Inherit: Same as input  ParamDataTypeStr=Inherit: Same as input
  Logical Operator : Logic  Operator=NOT  AllPortsSameDT=off  OutDataTypeStr=boolean
  Logical Operator5 : Logic  AllPortsSameDT=off  OutDataTypeStr=boolean
  MATLAB Function : MATLAB Function  TreatAsAtomicUnit=on
  MATLAB Function1 : MATLAB Function  TreatAsAtomicUnit=on
  Memory : Memory  InitialCondition=1
  Memory1 : Memory  InitialCondition=1
  Mux{,1..2,5,8} (5 alike) : Mux  Inputs=2
  Polar to Cartesian : simulink_extras/Transformations/Polar to Cartesian
  Real-Imag to Complex1 : RealImagToComplex
  Real-Imag to Complex4 : RealImagToComplex
  Relay : Relay  OnSwitchValue=0.9  OffSwitchValue=0.85
  Saturation : Saturate  UpperLimit=Ilim  LowerLimit=0
  Saturation1 : Saturate  UpperLimit=1  LowerLimit=0.1
  Scope : Scope
  Scope1 : Scope  NumInputPorts=2
  Scope2 : Scope  NumInputPorts=3
  Scope3 : Scope  NumInputPorts=2
  Scope4 : Scope
  Scope5 : Scope
  Static : Gain  Gain=1/(0.1*1i)  SaturateOnIntegerOverflow=on  OutDataTypeStr=Inherit: Same as input  ParamDataTypeStr=Inherit: Same as input
  Sum1 : Sum  Inputs=+-
  Sum2 : Sum  Inputs=+-
  Sum3 : Sum  Inputs=++++
  Switch1 : Switch  Threshold=tdist - 0.4  SaturateOnIntegerOverflow=off  InputSameDT=off
  Switch4 : Switch  Threshold=0.5  SaturateOnIntegerOverflow=off  InputSameDT=off
  Switch5 : Switch  Threshold=tdist - 0.5  SaturateOnIntegerOverflow=off  InputSameDT=off
  Terminator : Terminator
  Transfer Fcn1 : TransferFcn  Numerator=[2*pi*100]  Denominator=[1 2*pi*100]
  Transfer Fcn2 : TransferFcn  Numerator=[2*pi*200]  Denominator=[1 2*pi*200]
  Transfer Fcn3 : TransferFcn  Numerator=[2*pi*100]  Denominator=[1 2*pi*100]
  Transfer Fcn4 : TransferFcn  Numerator=[2*pi*30]  Denominator=[1 2*pi*30]
  Transfer Fcn5 : TransferFcn  Denominator=[0.01 1]
  Transfer Fcn6 : TransferFcn  Denominator=[0.01 1]
  Transfer Fcn7 : TransferFcn  Denominator=[0.01 1]
  Transfer Fcn9 : TransferFcn  Numerator=[2*pi*200]  Denominator=[1 2*pi*200]
  i ref : Outport
  wires:
  vref/1 -> Demux4/1, Sum1/1
  Demux1/2 -> Transfer Fcn3/1
  Demux/1 -> Cartesian to Polar/1
  Mux8/1 -> Sum1/2, Kp3/1
  Cartesian to Polar/2 -> Polar to Cartesian/2
  Demux/2 -> Cartesian to Polar/2
  Bypass startup/1 -> Polar to Cartesian/1  "Iamp"
  Integrator1/1 -> Sum3/2
  Mux1/1 -> Kp5/1
  Kp1/1 -> Integrator1/1
  Transfer Fcn1/1 -> Mux1/1
  Kp2/1 -> Sum3/1
  Transfer Fcn3/1 -> Mux1/2
  If/1 -> Demux1/1
  Demux1/1 -> Transfer Fcn1/1
  Kp5/1 -> Sum3/3
  Mux2/1 -> Demux/1
  Sum1/1 -> Kp2/1, Scope/1, Kp1/1
  Polar to Cartesian/1 -> Mux/1
  Polar to Cartesian/2 -> Mux/2
  Mux/1 -> i ref/1
  Cartesian to Polar/1 -> [iref_mag], Scope1/1, Saturation/1, Bypass startup/3  "Iref"
  Transfer Fcn2/1 -> Mux8/2
  Transfer Fcn9/1 -> Mux8/1
  Demux3/2 -> Transfer Fcn2/1
  Demux3/1 -> Transfer Fcn9/1
  Kp3/1 -> Sum3/4
  Cartesian to Polar1/2 -> Terminator/1
  Cartesian to Polar1/1 -> Transfer Fcn4/1
  Demux2/2 -> Cartesian to Polar1/2
  Demux2/1 -> Cartesian to Polar1/1
  v/1 -> Demux3/1, Demux2/1, Demux5/1
  Transfer Fcn4/1 -> [Vmag]
  Static/1 -> Complex to Real-Imag/1
  Complex to Real-Imag/2 -> Mux2/2
  [iref_mag] -> Divide/1
  Constant3/1 -> Switch4/3
  [v_pha_va] -> Divide1/2
  Transfer Fcn5/1 -> Switch4/1, Scope3/1
  [FRT] -> Switch4/2
  [iref_sat_mag] -> Divide/2
  Saturation1/1 -> Scope3/2, Divide1/1  "mu"
  [vref_pha] -> Sum2/1
  Divide/1 -> Transfer Fcn5/1
  Complex to Real-Imag/1 -> Mux2/1
  Switch4/1 -> Saturation1/1
  Sum2/1 -> Static/1
  Saturation/1 -> Scope1/2, [iref_sat_mag], Bypass startup/1  "Iamp"
  Clock1/1 -> Bypass startup/2
  Demux4/2 -> Real-Imag to Complex1/2
  Demux4/1 -> Real-Imag to Complex1/1
  Real-Imag to Complex1/1 -> [vref_pha]
  Real-Imag to Complex4/1 -> [v_pha_va]
  Demux5/1 -> Transfer Fcn7/1
  Demux5/2 -> Transfer Fcn6/1
  Transfer Fcn7/1 -> Real-Imag to Complex4/1
  Transfer Fcn6/1 -> Real-Imag to Complex4/2
  Constant1/1 -> Switch1/3
  Clock3/1 -> Switch1/2
  Switch1/1 -> Mux5/2
  Constant6/1 -> Switch5/3
  Data Type Conversion/1 -> Mux5/1
  Logical Operator/1 -> Scope2/1, Edge Detector/1, Logical Operator5/2
  Clock4/1 -> Switch5/2
  MATLAB Function1/1(output) -> Logical Operator/1, Memory1/1, Scope5/1
  MATLAB Function/1(y) -> Scope2/2, Logical Operator5/1
  Edge Detector/1 -> Data Type Conversion/1
  Switch5/1 -> [FRT], Scope2/3
  Mux5/1 -> MATLAB Function/1(u)
  [Vmag] -> Relay/1, Scope4/1, Memory/1, MATLAB Function1/1(input)
  Logical Operator5/1 -> Switch5/1
  Constant/1 -> Switch1/1
  Divide1/1 -> Sum2/2
  Memory/1 -> MATLAB Function1/4(prevIn)
  Constant4/1 -> MATLAB Function1/2(upper)
  Constant2/1 -> MATLAB Function1/3(lower)
  Memory1/1 -> MATLAB Function1/5(preOut)

== system B2_IEEE_13_bus/DER aggregation/Inverter Control/Volt T ==
  abc : Inport
  In2 : Inport  Port=2
  Demux : Demux  Outputs=3
  Mux1 : Mux  Inputs=2
  Subsystem : Subsystem
  Terminator2 : Terminator
  abc to Alpha-Beta-Zero : spsabctoAlphaBetaZeroLib/abc to Alpha-Beta-Zero
  dq : Outport
  wires:
  Subsystem/1(dq) -> dq/1
  abc to Alpha-Beta-Zero/1 -> Demux/1
  Demux/3 -> Terminator2/1
  Demux/1 -> Mux1/1
  Demux/2 -> Mux1/2
  abc/1 -> abc to Alpha-Beta-Zero/1
  Mux1/1 -> Subsystem/1(albe)
  In2/1 -> Subsystem/2(wt)

== system B2_IEEE_13_bus/DER aggregation/Inverter Control/Curr T/Subsystem ==
  note: d = al*cos(wt) + be*sin(wt)
  note: q = -al*sin(wt) + be*cos(wt)
  albe : Inport
  wt : Inport  Port=2
  Fcn : Fcn  Expr=u[1]*cos(u[3]) + u[2]*sin(u[3])
  Fcn1 : Fcn  Expr=-u[1]*sin(u[3]) + u[2]*cos(u[3])
  Mux : Mux  Inputs=2
  Mux2 : Mux  Inputs=[2 1]
  Mux3 : Mux  Inputs=[2 1]
  dq : Outport
  wires:
  Fcn1/1 -> Mux/2
  wt/1 -> Mux2/2, Mux3/2
  Fcn/1 -> Mux/1
  Mux/1 -> dq/1
  albe/1 -> Mux2/1, Mux3/1
  Mux2/1 -> Fcn/1
  Mux3/1 -> Fcn1/1

== system B2_IEEE_13_bus/DER aggregation/Inverter Control/Curr in T/Subsystem ==
  note: d = al*cos(wt) + be*sin(wt)
  note: q = -al*sin(wt) + be*cos(wt)
  albe : Inport
  wt : Inport  Port=2
  Fcn : Fcn  Expr=u[1]*cos(u[3]) + u[2]*sin(u[3])
  Fcn1 : Fcn  Expr=-u[1]*sin(u[3]) + u[2]*cos(u[3])
  Mux : Mux  Inputs=2
  Mux2 : Mux  Inputs=[2 1]
  Mux3 : Mux  Inputs=[2 1]
  dq : Outport
  wires:
  Fcn1/1 -> Mux/2
  wt/1 -> Mux2/2, Mux3/2
  Fcn/1 -> Mux/1
  Mux/1 -> dq/1
  albe/1 -> Mux2/1, Mux3/1
  Mux2/1 -> Fcn/1
  Mux3/1 -> Fcn1/1

== system B2_IEEE_13_bus/DER aggregation/Inverter Control/Volt T/Subsystem ==
  note: q = -al*sin(wt) + be*cos(wt)
  note: d = al*cos(wt) + be*sin(wt)
  albe : Inport
  wt : Inport  Port=2
  Fcn : Fcn  Expr=u[1]*cos(u[3]) + u[2]*sin(u[3])
  Fcn1 : Fcn  Expr=-u[1]*sin(u[3]) + u[2]*cos(u[3])
  Mux : Mux  Inputs=2
  Mux2 : Mux  Inputs=[2 1]
  Mux3 : Mux  Inputs=[2 1]
  dq : Outport
  wires:
  Mux3/1 -> Fcn1/1
  Mux2/1 -> Fcn/1
  albe/1 -> Mux3/1, Mux2/1
  Mux/1 -> dq/1
  Fcn/1 -> Mux/1
  wt/1 -> Mux3/2, Mux2/2
  Fcn1/1 -> Mux/2

== matlab function B2_IEEE_13_bus/DER aggregation/Inverter Control/Volt Ctrl/MATLAB Function1 ==
  settings: updateMethod=DISCRETE
  data: input input; output output boolean; upper input; lower input; prevIn input; preOut input boolean
function output = HC(input, upper, lower, prevIn, preOut)
% newHysteresisComparator
%
% input         - Current input signal
% upper         - Upper threshold for triggering high output
% lower         - Lower threshold for triggering low output
% prev          - Previous output state
%
% output        - Current output state

    % Initial output state
    if isempty(preOut)
        preOut = true; % Default previous output state
    end

    % Hysteresis logic
    if input > upper
        output = true; % Output is high if input exceeds upper threshold
    elseif input < lower
        output = false; % Output is low if input falls below lower threshold
    else
        if prevIn >= lower && prevIn <= upper
            output = preOut;
        else
            output = ~logical(preOut);
        end
    end
end

== matlab function B2_IEEE_13_bus/DER aggregation/Inverter Control/Volt Ctrl/MATLAB Function ==
  settings: updateMethod=DISCRETE
  data: u input; y output
function y = fcn(u)
persistent x;
if isempty (x)
    x = 1;
end

if u(2) == 1
    if u(1) == 1
        x = 0;
    end
else
    x = 1;
end
y = x;
